simulink model "yaw_accn"  (R2015a)
settings: Solver=ode45  StartTime=0.0  StopTime=12  RelTol=1e-3
settings Model: Creator=BML  LastModifiedBy=BML

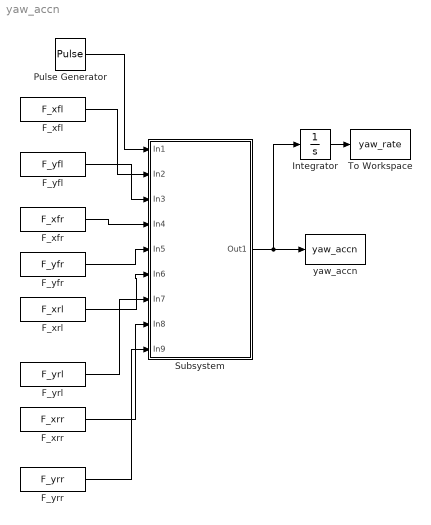
== system yaw_accn ==
  F_xfl : FromWorkspace  VariableName=F_xfl  SampleTime=0
  F_xfr : FromWorkspace  VariableName=F_xfr  SampleTime=0
  F_xrl : FromWorkspace  VariableName=F_xrl  SampleTime=0
  F_xrr : FromWorkspace  VariableName=F_xrr  SampleTime=0
  F_yfl : FromWorkspace  VariableName=F_yfl  SampleTime=0
  F_yfr : FromWorkspace  VariableName=F_yfr  SampleTime=0
  F_yrl : FromWorkspace  VariableName=F_yrl  SampleTime=0
  F_yrr : FromWorkspace  VariableName=F_yrr  SampleTime=0
  Integrator : Integrator
  Pulse Generator : DiscretePulseGenerator  PulseType=Time based  Amplitude=0  Period=8  PulseWidth=5  PhaseDelay=3
  Subsystem : Subsystem
  To Workspace : ToWorkspace  VariableName=yaw_rate  SaveFormat=Timeseries  SampleTime=-1
  yaw_accn : ToWorkspace  VariableName=yaw_accn  SaveFormat=Timeseries  SampleTime=-1
  wires:
  Pulse Generator/1 -> Subsystem/1(In1)
  F_xfl/1 -> Subsystem/2(In2)
  F_yfl/1 -> Subsystem/3(In3)
  F_xfr/1 -> Subsystem/4(In4)
  F_yfr/1 -> Subsystem/5(In5)
  F_xrl/1 -> Subsystem/6(In6)
  F_yrl/1 -> Subsystem/7(In7)
  F_xrr/1 -> Subsystem/8(In8)
  F_yrr/1 -> Subsystem/9(In9)
  Subsystem/1(Out1) -> Integrator/1, yaw_accn/1
  Integrator/1 -> To Workspace/1

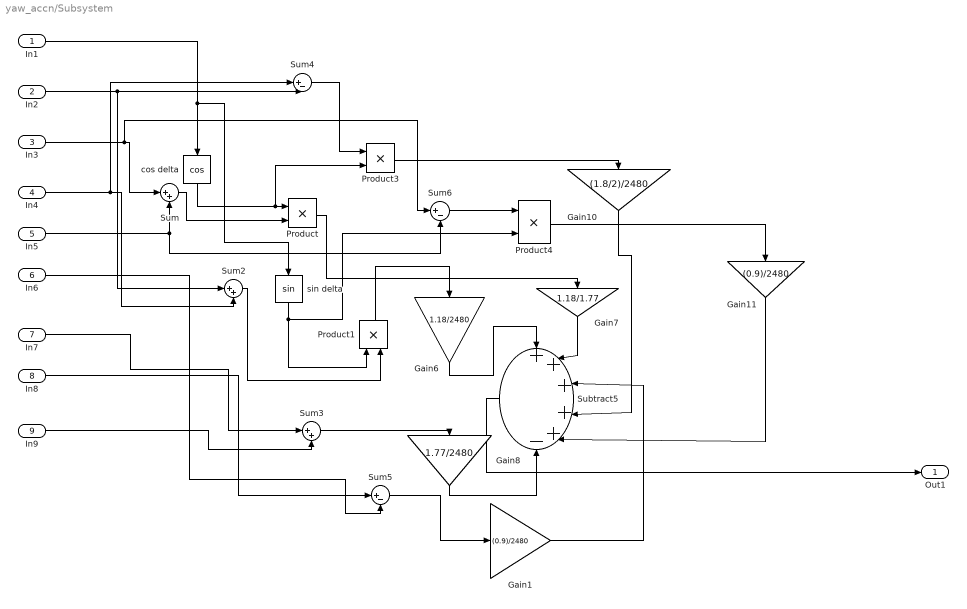
== system yaw_accn/Subsystem ==
  In1 : Inport
  In2 : Inport  Port=2
  In3 : Inport  Port=3
  In4 : Inport  Port=4
  In5 : Inport  Port=5
  In6 : Inport  Port=6
  In7 : Inport  Port=7
  In8 : Inport  Port=8
  In9 : Inport  Port=9
  Gain1 : Gain  Gain=(0.9)/2480
  Gain10 : Gain  Gain=(1.8/2)/2480
  Gain11 : Gain  Gain=(0.9)/2480
  Gain6 : Gain  Gain=1.18/2480
  Gain7 : Gain  Gain=1.18/1.77
  Gain8 : Gain  Gain=1.77/2480
  Product{,1,3..4} (4 alike) : Product
  Subtract5 : Sum  Inputs=+++++-
  Sum : Sum  Inputs=|++
  Sum2 : Sum  Inputs=|++
  Sum3 : Sum  Inputs=|++
  Sum4 : Sum  Inputs=|+-
  Sum5 : Sum  Inputs=|+-
  Sum6 : Sum  Inputs=|+-
  cos delta : Trigonometry  Operator=cos
  "sin delta " : Trigonometry
  Out1 : Outport
  wires:
  Sum4/1 -> Product3/1
  In1/1 -> "sin delta "/1, cos delta/1
  In7/1 -> Sum3/1
  Product3/1 -> Gain10/1
  Gain10/1 -> Subtract5/4
  In8/1 -> Sum5/1
  In3/1 -> Sum6/1, Sum/1
  Gain11/1 -> Subtract5/5
  In9/1 -> Sum3/2
  In6/1 -> Sum5/2
  "sin delta "/1 -> Product4/2, Product1/1
  cos delta/1 -> Product3/2, Product/1
  Gain7/1 -> Subtract5/2
  In5/1 -> Sum6/2, Sum/2
  Gain6/1 -> Subtract5/1
  Gain8/1 -> Subtract5/6
  Product/1 -> Gain7/1
  In2/1 -> Sum2/1, Sum4/2
  Product1/1 -> Gain6/1
  Sum3/1 -> Gain8/1
  Sum/1 -> Product/2
  Sum2/1 -> Product1/2
  In4/1 -> Sum4/1, Sum2/2
  Sum6/1 -> Product4/1
  Subtract5/1 -> Out1/1
  Sum5/1 -> Gain1/1
  Gain1/1 -> Subtract5/3
  Product4/1 -> Gain11/1
